simulink model "Lab_5_ex12"  (R2021b)
settings: Solver=VariableStepAuto  StartTime=0.0  StopTime=10.0  RelTol=1e-3
values from neighbouring files (symbols this model uses):
  A_c = double(A_c)    [main.m]
  A_o = double(A_o)    [main.m]
  B_c = double(B_c)    [main.m]
  B_o = double(B_o)    [main.m]
  C_c = double(C_c)    [main.m]
  C_o = double(C_o)    [main.m]
settings Model: Creator=Rares  LastModifiedBy=Rares

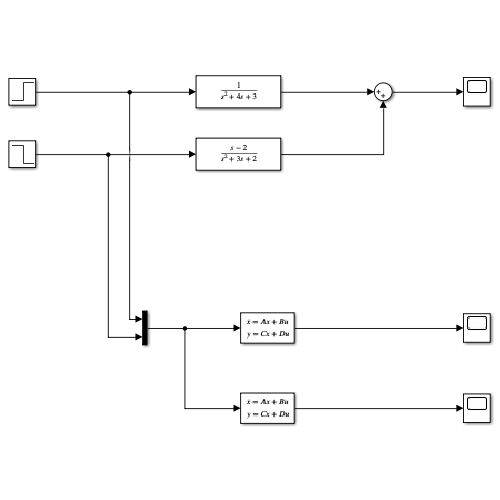
[thumbnail: Simulink's stored preview of the top-level diagram]
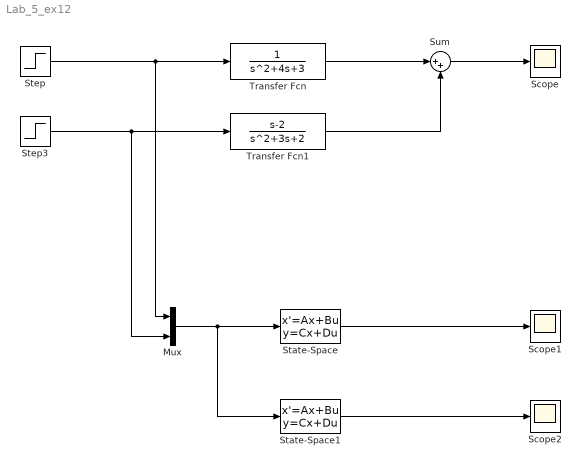
== system Lab_5_ex12 ==
  Mux : Mux  Inputs=2
  Scope : Scope
  Scope1 : Scope
  Scope2 : Scope
  State-Space : StateSpace  A=A_c  B=B_c  C=C_c  D=[0 0]  InitialCondition=0
  State-Space1 : StateSpace  A=A_o  B=B_o  C=C_o  D=[0 0]  InitialCondition=0
  Step : Step  Time=0  SampleTime=0
  Step3 : Step  Time=0  After=-2  SampleTime=0
  Sum : Sum  Inputs=|++
  Transfer Fcn : TransferFcn  Denominator=[1 4 3]
  Transfer Fcn1 : TransferFcn  Numerator=[1 -2]  Denominator=[1 3 2]
  wires:
  Step/1 -> Mux/1, Transfer Fcn/1
  Step3/1 -> Transfer Fcn1/1, Mux/2
  Transfer Fcn1/1 -> Sum/2
  Transfer Fcn/1 -> Sum/1
  Sum/1 -> Scope/1
  Mux/1 -> State-Space1/1, State-Space/1
  State-Space/1 -> Scope1/1
  State-Space1/1 -> Scope2/1
